simulink subsystem "getGyroDataNew"  (R2024a)
settings: Solver=VariableStepAuto  StartTime=0.0  StopTime=10.0  RelTol=1e-3
undefined symbols (not defined in the file or in its folder): bits, measRate
libraries: stm32blockslib x7
settings Model: Creator=Peter  LastModifiedBy=Peter

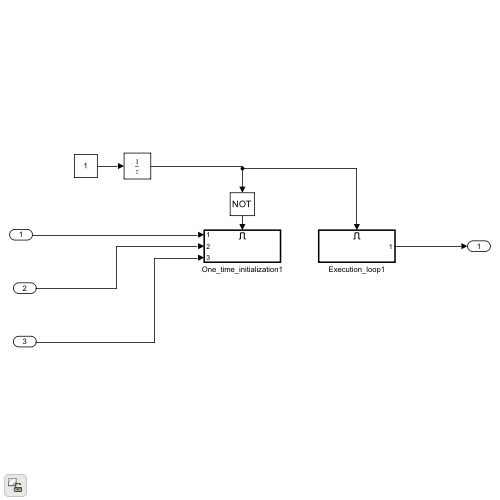
[thumbnail: Simulink's stored preview of the top-level diagram]
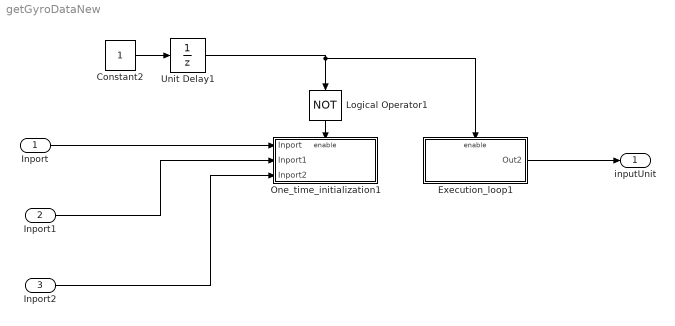
== system getGyroDataNew ==
  Inport : Inport
  Inport1 : Inport  Port=2
  Inport2 : Inport  Port=3
  Constant2 : Constant  OutDataTypeStr=boolean  SampleTime=measRate
  Execution_loop1 : Subsystem  TreatAsAtomicUnit=on
  Logical Operator1 : Logic  Operator=NOT  AllPortsSameDT=off  OutDataTypeStr=boolean
  One_time_initialization1 : Subsystem  TreatAsAtomicUnit=on
  Unit Delay1 : UnitDelay  SampleTime=-1  HasFrameUpgradeWarning=on
  inputUnit : Outport
  wires:
  Inport1/1 -> One_time_initialization1/2(Inport1)
  Inport2/1 -> One_time_initialization1/3(Inport2)
  Unit Delay1/1 -> Logical Operator1/1, Execution_loop1/Enable
  Logical Operator1/1 -> One_time_initialization1/Enable
  Constant2/1 -> Unit Delay1/1
  Inport/1 -> One_time_initialization1/1(Inport)
  Execution_loop1/1(Out2) -> inputUnit/1

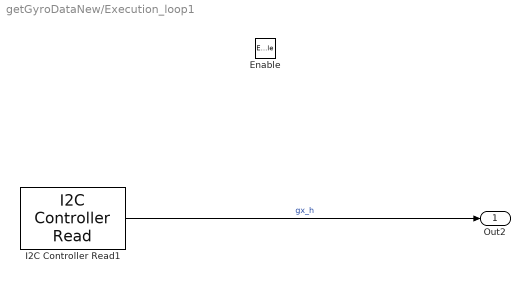
== system getGyroDataNew/Execution_loop1 ==
  Enable : EnablePort
  I2C Controller Read1 : stm32blockslib/I2C Controller Read  Priority=-1  I2CModule=I2C2  Mode=Controller  AddressingMode=7-bits  PeripheralByteOrder=LittleEndian  OwnPeripheralAddress=uint8(170)  PeripheralAddressVia=Dialog  PeripheralAddress=hex2dec('68')  RegisterAddressMode=on  RegisterAddressVia=Dialog  RegisterAddress=uint8(hex2dec('1D'))  RepeatedStart=off  NoAck=off  OutputStatus=off  BlockMode=Receive  DataType=uint8  DataLength=6  Timeout=0.001  SampleTime=inf
      settings: LibrarySourceBlock=stm32f7xxblockslib/I2C Controller Read
  Out2 : Outport  VectorParamsAs1DForOutWhenUnconnected=off
  wires:
  I2C Controller Read1/1 -> Out2/1  "gx_h"

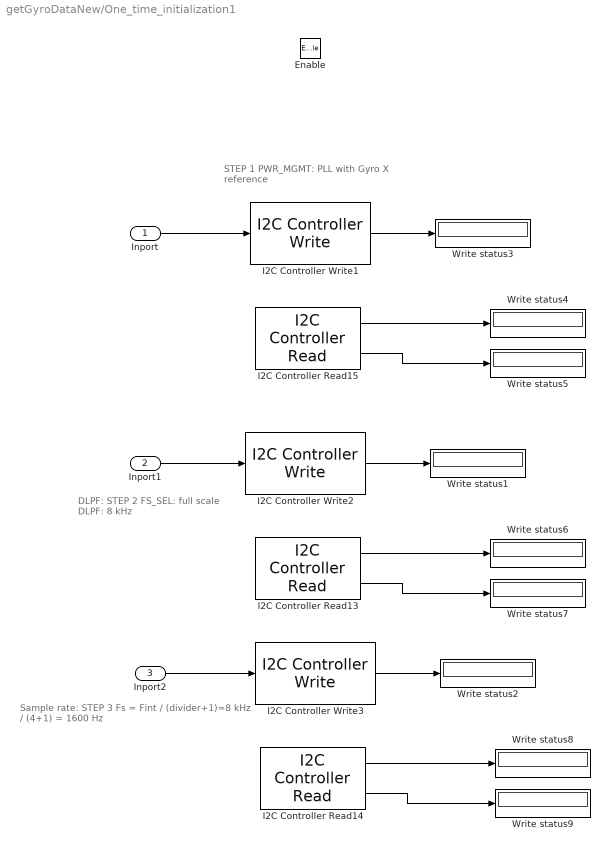
== system getGyroDataNew/One_time_initialization1 ==
  note: DLPF: STEP 2
      | FS_SEL: full scale
      | DLPF: 8 kHz
  note: STEP 1
      | PWR_MGMT: PLL with Gyro X reference
  note: Sample rate: STEP 3
      | Fs = Fint / (divider+1)=8 kHz / (4+1) = 1600 Hz
  Inport : Inport
  Inport1 : Inport  Port=2
  Inport2 : Inport  Port=3
  Enable : EnablePort
  I2C Controller Read13 : stm32blockslib/I2C Controller Read  Priority=-3  I2CModule=I2C2  Mode=Controller  AddressingMode=7-bits  PeripheralByteOrder=LittleEndian  OwnPeripheralAddress=uint8(170)  PeripheralAddressVia=Dialog  PeripheralAddress=hex2dec('68')  RegisterAddressMode=on  RegisterAddressVia=Dialog  RegisterAddress=uint8(hex2dec('16'))  RepeatedStart=off  NoAck=off  OutputStatus=on  BlockMode=Receive  DataType=uint8  DataLength=1  Timeout=0.001  SampleTime=inf
      settings: LibrarySourceBlock=stm32f7xxblockslib/I2C Controller Read
  I2C Controller Read14 : stm32blockslib/I2C Controller Read  Priority=-1  I2CModule=I2C2  Mode=Controller  AddressingMode=7-bits  PeripheralByteOrder=LittleEndian  OwnPeripheralAddress=uint8(170)  PeripheralAddressVia=Dialog  PeripheralAddress=hex2dec('68')  RegisterAddressMode=on  RegisterAddressVia=Dialog  RegisterAddress=uint8(hex2dec('15'))  RepeatedStart=off  NoAck=off  OutputStatus=on  BlockMode=Receive  DataType=uint8  DataLength=1  Timeout=0.001  SampleTime=inf
      settings: LibrarySourceBlock=stm32f7xxblockslib/I2C Controller Read
  I2C Controller Read15 : stm32blockslib/I2C Controller Read  Priority=-5  I2CModule=I2C2  Mode=Controller  AddressingMode=7-bits  PeripheralByteOrder=LittleEndian  OwnPeripheralAddress=uint8(170)  PeripheralAddressVia=Dialog  PeripheralAddress=hex2dec('68')  RegisterAddressMode=on  RegisterAddressVia=Dialog  RegisterAddress=uint8(hex2dec('3E'))  RepeatedStart=off  NoAck=off  OutputStatus=on  BlockMode=Receive  DataType=uint8  DataLength=1  Timeout=0.001  SampleTime=inf
      settings: LibrarySourceBlock=stm32f7xxblockslib/I2C Controller Read
  I2C Controller Write1 : stm32blockslib/I2C Controller Write  Priority=-6  I2CModule=I2C2  Mode=Controller  AddressingMode=7-bits  PeripheralByteOrder=LittleEndian  OwnPeripheralAddress=uint8(170)  PeripheralAddressVia=Dialog  PeripheralAddress=hex2dec('68')  RegisterAddressMode=on  RegisterAddressVia=Dialog  RegisterAddress=uint8(hex2dec('3E'))  RepeatedStart=off  NoAck=off  OutputStatus=on  BlockMode=Transmit  DataType=uint8  DataLength=1  Timeout=0.001  SampleTime=-1
      settings: LibrarySourceBlock=stm32f7xxblockslib/I2C Controller Write
  I2C Controller Write2 : stm32blockslib/I2C Controller Write  Priority=-4  I2CModule=I2C2  Mode=Controller  AddressingMode=7-bits  PeripheralByteOrder=LittleEndian  OwnPeripheralAddress=uint8(170)  PeripheralAddressVia=Dialog  PeripheralAddress=hex2dec('68')  RegisterAddressMode=on  RegisterAddressVia=Dialog  RegisterAddress=uint8(hex2dec('16'))  RepeatedStart=off  NoAck=off  OutputStatus=on  BlockMode=Transmit  DataType=uint8  DataLength=1  Timeout=0.001  SampleTime=-1
      settings: LibrarySourceBlock=stm32f7xxblockslib/I2C Controller Write
  I2C Controller Write3 : stm32blockslib/I2C Controller Write  Priority=-2  I2CModule=I2C2  Mode=Controller  AddressingMode=7-bits  PeripheralByteOrder=LittleEndian  OwnPeripheralAddress=uint8(170)  PeripheralAddressVia=Dialog  PeripheralAddress=hex2dec('68')  RegisterAddressMode=on  RegisterAddressVia=Dialog  RegisterAddress=uint8(hex2dec('15'))  RepeatedStart=off  NoAck=off  OutputStatus=on  BlockMode=Transmit  DataType=uint8  DataLength=1  Timeout=0.001  SampleTime=-1
      settings: LibrarySourceBlock=stm32f7xxblockslib/I2C Controller Write
  Write status{1..9} (9 alike) : Display
      settings: Format=hex (Stored Integer)
  wires:
  I2C Controller Read14/1 -> Write status8/1
  I2C Controller Write1/1 -> Write status3/1
  I2C Controller Write3/1 -> Write status2/1
  I2C Controller Read13/1 -> Write status6/1
  I2C Controller Write2/1 -> Write status1/1
  I2C Controller Read13/2 -> Write status7/1
  Inport1/1 -> I2C Controller Write2/1
  I2C Controller Read14/2 -> Write status9/1
  I2C Controller Read15/1 -> Write status4/1
  Inport/1 -> I2C Controller Write1/1
  I2C Controller Read15/2 -> Write status5/1
  Inport2/1 -> I2C Controller Write3/1
